simulink model "impedanceControl_phasePWM_test_R2017b"  (Simulink 9.0)
settings: Solver=FixedStepDiscrete  StartTime=0.0  StopTime=Config.SIMULATION_TIME  FixedStep=Config.Ts  RelTol=1e-3  EnableMultiTasking=on
InitFcn:
  | cd(fileparts(which(bdroot)));
  | initImpedanceControl_current_only;
StopFcn:
  | cd(fileparts(which(bdroot)));
  | stopImpedanceControl;
undefined symbols (not defined in the file or in its folder): Config, CONST_SETPOINT, CURRENT_IN_MILLI_AMPS, ELEC_TO_ROTOR_PHASE, MOVE_SELECTOR
libraries: WBToolboxLibrary x9, simulink x1
settings Model: SuppressorTable=22 serialization::archive 11 0 6 0 0 0 0 0  Creator=daniele  LastModifiedBy=nunoguedelha
settings DataIOCC: LimitDataPoints=on
settings DebuggingCC: UnderspecifiedInitializationDetection=Simplified  MergeDetectMultiDrivingBlocksExec=error  SolverPrmCheckMsg=warning  MultiTaskDSMMsg=warning  MultiTaskCondExecSysMsg=none  AllowSymbolicDim=off  StrictBusMsg=ErrorOnBusTreatedAsVector
settings GRTTargetCC: GeneratePreprocessorConditionals=Disable all

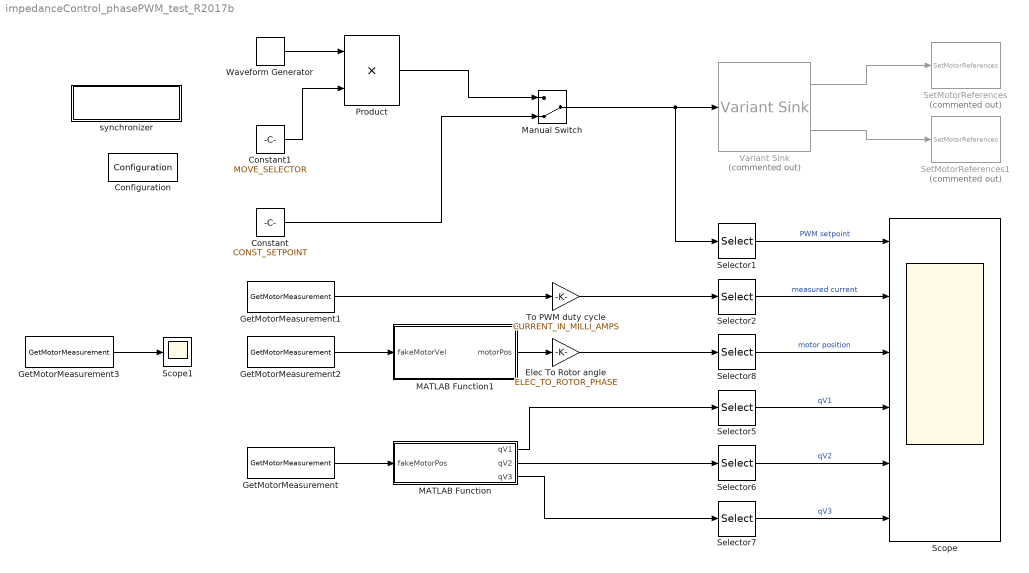
== system impedanceControl_phasePWM_test_R2017b ==
  Configuration : WBToolboxLibrary/Utilities/Configuration  ConfigSource=Workspace  ConfigObject='WBTConfigRobot'
      settings: SourceProductName=WholeBodyToolbox
  Constant : Constant  Value=CONST_SETPOINT
  Constant1 : Constant  Value=MOVE_SELECTOR
  Elec To Rotor angle : Gain  Gain=ELEC_TO_ROTOR_PHASE
  GetMotorMeasurement : WBToolboxLibrary/States/GetMotorMeasurement  measuredType=Motor Position
      settings: SourceProductName=WholeBodyToolbox
  GetMotorMeasurement1 : WBToolboxLibrary/States/GetMotorMeasurement  measuredType=Motor Current
      settings: SourceProductName=WholeBodyToolbox
  GetMotorMeasurement2 : WBToolboxLibrary/States/GetMotorMeasurement  measuredType=Motor Velocity
      settings: SourceProductName=WholeBodyToolbox
  GetMotorMeasurement3 : WBToolboxLibrary/States/GetMotorMeasurement  measuredType=Motor PWM
      settings: SourceProductName=WholeBodyToolbox
  MATLAB Function : MATLAB Function  TreatAsAtomicUnit=on
  MATLAB Function1 : MATLAB Function  TreatAsAtomicUnit=on
  Manual Switch : ManualSwitch  CurrentSetting=0
  Product : Product  Inputs=**
  Scope : Scope  NumInputPorts=6
  Scope1 : Scope
  Selector{1..2,5..8} (6 alike) : Selector  InputPortWidth=ROBOT_DOF  IndexOptions=Index vector (dialog)  Indices=JOINTS_TO_PLOT  OutputSizes=1
  SetMotorReferences : WBToolboxLibrary/Actuators/SetMotorReferences  Commented=on  controlType=PWM
      settings: SourceProductName=WholeBodyToolbox
  SetMotorReferences1 : WBToolboxLibrary/Actuators/SetMotorReferences  Commented=on  controlType=Current
      settings: SourceProductName=WholeBodyToolbox
  To PWM duty cycle : Gain  Gain=CURRENT_IN_MILLI_AMPS
  Variant Sink : VariantSink  Commented=on  VariantControls=DataTag0
  Waveform Generator : simulink/Sources/Waveform Generator  OutMin=[]  OutMax=[]  OutDataTypeStr=double  SelectedSignal=2  Signals=sin('Amplitude',AMPLS_SETPOINT_SCALAR,'Frequency',FREQS_SETPOINT_SCALAR*2*pi,'Phase',0)#square('Amplitude',AMPLS_SETPOINT_SCALAR,'Frequency',FREQS_SETPOINT_SCALAR*2*pi,'Phase',0)  BlockNames=MultiportSwitch_3178556914cb42a#MultiportSwitch_475149221586492  SampleTime=Config.Ts
      settings: SourceProductName=Simulink
  synchronizer : Subsystem
      mask Display: disp('SYNCHRONIZER')
  wires:
  MATLAB Function1/1(motorPos) -> Elec To Rotor angle/1
  Selector1/1 -> Scope/1  "PWM setpoint"
  Selector2/1 -> Scope/2  "measured current"
  Selector8/1 -> Scope/3  "motor position"
  GetMotorMeasurement1/1 -> To PWM duty cycle/1
  Product/1 -> Manual Switch/1
  Constant/1 -> Manual Switch/2
  Manual Switch/1 -> Variant Sink/1, Selector1/1
  Variant Sink/1 -> SetMotorReferences/1
  Variant Sink/2 -> SetMotorReferences1/1
  Waveform Generator/1 -> Product/1
  Constant1/1 -> Product/2
  Selector5/1 -> Scope/4  "qV1"
  Selector6/1 -> Scope/5  "qV2"
  MATLAB Function/1(qV1) -> Selector5/1
  GetMotorMeasurement2/1 -> MATLAB Function1/1(fakeMotorVel)
  GetMotorMeasurement/1 -> MATLAB Function/1(fakeMotorPos)
  MATLAB Function/3(qV3) -> Selector7/1
  Elec To Rotor angle/1 -> Selector8/1
  Selector7/1 -> Scope/6  "qV3"
  MATLAB Function/2(qV2) -> Selector6/1
  To PWM duty cycle/1 -> Selector2/1
  GetMotorMeasurement3/1 -> Scope1/1

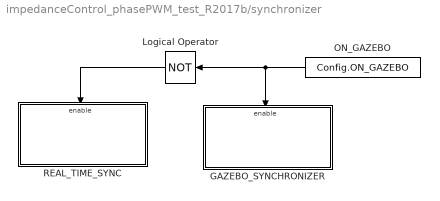
== system impedanceControl_phasePWM_test_R2017b/synchronizer ==
  GAZEBO_SYNCHRONIZER : Subsystem
  Logical Operator : Logic  Operator=NOT  AllPortsSameDT=off  OutDataTypeStr=boolean
  "ON_GAZEBO " : Constant  Value=Config.ON_GAZEBO
  REAL_TIME_SYNC : Subsystem
  wires:
  Logical Operator/1 -> REAL_TIME_SYNC/Enable
  "ON_GAZEBO "/1 -> GAZEBO_SYNCHRONIZER/Enable, Logical Operator/1

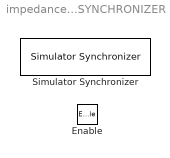
== system impedanceControl_phasePWM_test_R2017b/synchronizer/GAZEBO_SYNCHRONIZER ==
  Enable : EnablePort
  Simulator Synchronizer : WBToolboxLibrary/Utilities/Simulator Synchronizer  period=Config.Ts  serverPortName='/clock/rpc'  clientPortName='/WBT_synchronizer/rpc:o'
      settings: SourceProductName=WholeBodyToolbox

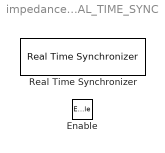
== system impedanceControl_phasePWM_test_R2017b/synchronizer/REAL_TIME_SYNC ==
  Enable : EnablePort
  Real Time Synchronizer : WBToolboxLibrary/Utilities/Real Time Synchronizer  period=Config.Ts
      settings: SourceProductName=WholeBodyToolbox

== matlab function MATLAB Function1 ==
  data: fakeMotorVel input double; motorPos output double
function motorPos = getElCyclePosition(fakeMotorVel)
% in the 2FOC, we logged the motor position (in degrees) in place of the motor velocity.
[~,motorPos] = motorYarpPos2motorfocPosUnits(fakeMotorVel);

== matlab function MATLAB Function ==
  data: fakeMotorPos input double size=1; qV1 output double size=1; qV2 output double size=1; qV3 output double size=1
function [qV1,qV2,qV3] = parseCurrents(fakeMotorPos)

% Convert to original format used in 2FOC code, sent by the CAN transmitter
qIaqIc = motorYarpPos2motorfocPosUnits(fakeMotorPos);

% Convert to signed hexadecimal
uqIaqIc = typecast(int32(qIaqIc),'uint32');

% Split qIa from qIc
qIaMask = hex2dec('0000FFFF');
qIcMask = hex2dec('FFFF0000');
uqIa = bitand(uqIaqIc,qIaMask);
uqIc = bitshift(bitand(uqIaqIc,qIcMask),-16);

qV1 = double(typecast(uint16(uqIa),'int16'));
qV3 = double(typecast(uint16(uqIc),'int16'));
qV2 = -qV1-qV3;
